simulink model "PID_SingleJoint"  (R2018b)
settings: Solver=FixedStepDiscrete  StartTime=0.0  StopTime=Inf  FixedStep=0.001  RelTol=1e-3  EnableMultiTasking=on
undefined symbols (not defined in the file): DiscIntNeverNeededParam, J1, J2, J3, J4, J5, J6, J7, Motor_Current, Motor_Position, Motor_Velocity, q, qd, Send_GUIdata, Tau
libraries: c280xlib x14, simulink x11, dspsrcs4 x6, idelinklib_common x1
(part 2 of 4)

== system PID_SingleJoint/DynamicsController/关节四正弦信号发生器 ==
  note: 0~60
  En : Inport
  q : Inport  Port=2
  Constant3 : Constant  Value=30
  Gain14 : Gain  Gain=pi/180
  Subsystem : Subsystem  mask(单关节正弦信号生产器){Freq=1/4, SimpleTime=0.001}
      mask prompts: Freq "正弦信号的频率(HZ)"; SimpleTime "正弦信号的采样时间(s)"
      mask help:
      | 采样频率不能过快，否则机械臂摆动频率也会变快，至少为1/4.
      | 采样时间只能是定时器步长的整数倍，否则会报错。
      mask Display:
      | color('red');
      | disp('单关节正弦信号发生器');
      | color('black');
      | port_label('input', 1, '外转子实际角度(rad)');
      | port_label('input', 2, '外转子正弦信号的幅值');
      | port_label('Enable','Enable')
      | port_label('output', 1, '外转子理想正弦信号');
      | port_label('output', 2, '外转子跟踪误差(rad)');
  qd : Outport
  e : Outport  Port=2
  wires:
  q/1 -> Subsystem/1(电机外转子 实际角度(rad))
  En/1 -> Subsystem/Enable
  Gain14/1 -> Subsystem/2(电机外转子 正弦信号的幅值)
  Subsystem/2(电机外转子 跟踪误差) -> e/1
  Constant3/1 -> Gain14/1
  Subsystem/1(外转子理想 正弦信号) -> qd/1

== system PID_SingleJoint/GetMotorData/CANA_284_24 ==
  note: 控制器接收ID:0x280+“ID”
  Subsystem1 : Subsystem
  eCAN Receive1 : c280xlib/eCAN Receive  chipFamily=C280x  useModule=eCAN_A  mailboxNo=24  messageID=hex2dec('284')  messageType=Standard (11-bit identifier)  sampleTime=-1  dataType=uint8  initValue=0  outputMessageLength=off  outputMessageTimeStamp=off  postInterrupt=off  interruptLine=0
      settings: SourceProductName=Embedded Coder Support Package for Texas Instruments C2000 Processors  SourceProductBaseCode=TIC2000
  wires:
  eCAN Receive1/2 -> Subsystem1/1(In1)
  eCAN Receive1/1 -> Subsystem1/Trigger

== system PID_SingleJoint/GetMotorData/CANA_285_25 ==
  note: 控制器接收ID:0x280+“ID”
  Subsystem : Subsystem
  eCAN Receive : c280xlib/eCAN Receive  chipFamily=C280x  useModule=eCAN_A  mailboxNo=25  messageID=hex2dec('285')  messageType=Standard (11-bit identifier)  sampleTime=-1  dataType=uint8  initValue=0  outputMessageLength=off  outputMessageTimeStamp=off  postInterrupt=off  interruptLine=0
      settings: SourceProductName=Embedded Coder Support Package for Texas Instruments C2000 Processors  SourceProductBaseCode=TIC2000
  wires:
  eCAN Receive/2 -> Subsystem/1(In1)
  eCAN Receive/1 -> Subsystem/Trigger

== system PID_SingleJoint/GetMotorData/CANA_286_26 ==
  note: 控制器接收ID:0x280+“ID”
  Subsystem : Subsystem
  eCAN Receive : c280xlib/eCAN Receive  chipFamily=C280x  useModule=eCAN_A  mailboxNo=26  messageID=hex2dec('286')  messageType=Standard (11-bit identifier)  sampleTime=-1  dataType=uint8  initValue=0  outputMessageLength=off  outputMessageTimeStamp=off  postInterrupt=off  interruptLine=0
      settings: SourceProductName=Embedded Coder Support Package for Texas Instruments C2000 Processors  SourceProductBaseCode=TIC2000
  wires:
  eCAN Receive/2 -> Subsystem/1(In1)
  eCAN Receive/1 -> Subsystem/Trigger

== system PID_SingleJoint/GetMotorData/CANB_281_21 ==
  note: 控制器接收ID:0x280+“ID”
  Subsystem : Subsystem
  eCAN Receive : c280xlib/eCAN Receive  chipFamily=C280x  useModule=eCAN_B  mailboxNo=21  messageID=hex2dec('281')  messageType=Standard (11-bit identifier)  sampleTime=-1  dataType=uint8  initValue=0  outputMessageLength=off  outputMessageTimeStamp=off  postInterrupt=off  interruptLine=0
      settings: SourceProductName=Embedded Coder Support Package for Texas Instruments C2000 Processors  SourceProductBaseCode=TIC2000
  wires:
  eCAN Receive/2 -> Subsystem/1(In1)
  eCAN Receive/1 -> Subsystem/Trigger

== system PID_SingleJoint/GetMotorData/CANB_282_22 ==
  note: 控制器接收ID:0x280+“ID”
  Subsystem : Subsystem
  eCAN Receive : c280xlib/eCAN Receive  chipFamily=C280x  useModule=eCAN_B  mailboxNo=22  messageID=hex2dec('282')  messageType=Standard (11-bit identifier)  sampleTime=-1  dataType=uint8  initValue=0  outputMessageLength=off  outputMessageTimeStamp=off  postInterrupt=off  interruptLine=0
      settings: SourceProductName=Embedded Coder Support Package for Texas Instruments C2000 Processors  SourceProductBaseCode=TIC2000
  wires:
  eCAN Receive/2 -> Subsystem/1(In1)
  eCAN Receive/1 -> Subsystem/Trigger

== system PID_SingleJoint/GetMotorData/CANB_283_23 ==
  note: 控制器接收ID:0x280+“ID”
  Subsystem : Subsystem
  eCAN Receive : c280xlib/eCAN Receive  chipFamily=C280x  useModule=eCAN_B  mailboxNo=23  messageID=hex2dec('283')  messageType=Standard (11-bit identifier)  sampleTime=-1  dataType=uint8  initValue=0  outputMessageLength=off  outputMessageTimeStamp=off  postInterrupt=off  interruptLine=0
      settings: SourceProductName=Embedded Coder Support Package for Texas Instruments C2000 Processors  SourceProductBaseCode=TIC2000
  wires:
  eCAN Receive/2 -> Subsystem/1(In1)
  eCAN Receive/1 -> Subsystem/Trigger

== system PID_SingleJoint/SendDataToGUI/  ==
  Enable : EnablePort
  Constant1 : Constant  Value=hex2dec('5a')  OutDataTypeStr=uint16
  Data Store Read4 : DataStoreRead  DataStoreName=Send_GUIdata
  Data Type Conversion12 : DataTypeConversion  OutDataTypeStr=uint16
  Demux : Demux  Outputs=18
  Mux : Mux  Inputs=20
  SCI Transmit : c280xlib/SCI Transmit  sciModule=A  dataHead=''  dataTail=''  postInterrupt=off  numFifo=1
      settings: SourceProductName=Embedded Coder Support Package for Texas Instruments C2000 Processors
  校验码填充 : Sum  Inputs=+++++++++++++++++++  AccumDataTypeStr=uint16
  wires:
  Demux/1 -> Mux/2, 校验码填充/2
  Mux/1 -> SCI Transmit/1
  Demux/3 -> 校验码填充/4, Mux/4
  Demux/14 -> 校验码填充/15, Mux/15
  Demux/9 -> 校验码填充/10, Mux/10
  Demux/5 -> Mux/6, 校验码填充/6
  Demux/2 -> 校验码填充/3, Mux/3
  Data Store Read4/1 -> Data Type Conversion12/1
  Demux/13 -> 校验码填充/14, Mux/14
  Demux/6 -> Mux/7, 校验码填充/7
  Demux/8 -> 校验码填充/9, Mux/9
  Demux/10 -> 校验码填充/11, Mux/11
  Demux/4 -> 校验码填充/5, Mux/5
  Demux/7 -> 校验码填充/8, Mux/8
  Demux/15 -> 校验码填充/16, Mux/16
  Demux/11 -> 校验码填充/12, Mux/12
  Demux/18 -> 校验码填充/19, Mux/19
  Demux/16 -> 校验码填充/17, Mux/17
  Constant1/1 -> 校验码填充/1, Mux/1
  Demux/17 -> 校验码填充/18, Mux/18
  校验码填充/1 -> Mux/20
  Demux/12 -> 校验码填充/13, Mux/13
  Data Type Conversion12/1 -> Demux/1

== system PID_SingleJoint/Subsystem/Model Header ==

== system PID_SingleJoint/Subsystem/Model Source ==

== system PID_SingleJoint/Subsystem/System Initialize ==

== system PID_SingleJoint/接收上位机的数据/Subsystem ==
  组号 : Inport
  数据 : Inport  Port=2
  Enable : EnablePort
  Joint1 : Subsystem  TreatAsAtomicUnit=on
  Joint2 : Subsystem  TreatAsAtomicUnit=on
  Joint3 : Subsystem  TreatAsAtomicUnit=on
  Joint4 : Subsystem  TreatAsAtomicUnit=on
  Joint5 : Subsystem  TreatAsAtomicUnit=on
  Joint6 : Subsystem  TreatAsAtomicUnit=on
  Joint7 : Subsystem  TreatAsAtomicUnit=on
  Switch Case : SwitchCase  CaseConditions={1 2 3 4 5 6 7}  ShowDefaultCase=off
  wires:
  数据/1 -> Joint7/1(Joint7), Joint5/1(Joint5), Joint4/1(Joint4), Joint3/1(Joint3), Joint2/1(Joint2), Joint1/1(Joint1), Joint6/1(Joint6)
  Switch Case/5 -> Joint5/Action
  Switch Case/6 -> Joint6/Action
  Switch Case/2 -> Joint2/Action
  Switch Case/1 -> Joint1/Action
  Switch Case/3 -> Joint3/Action
  Switch Case/4 -> Joint4/Action
  组号/1 -> Switch Case/1
  Switch Case/7 -> Joint7/Action

== system PID_SingleJoint/接收上位机的数据/获取用户命令 ==
  " " : c280xlib/SCI Receive  sciModule=A  dataHead=''  dataTail=''  dataType=uint16  dataDim=9  initValue=0  errOption=Output the last received value  errValue=0  sampleTime=-1  outputStatus=on  postInterrupt=off  numFifo=1
      settings: SourceProductName=Embedded Coder Support Package for Texas Instruments C2000 Processors  SourceProductBaseCode=TIC2000
  Constant : Constant  Value=false  OutDataTypeStr=boolean
  Constant1 : Constant  Value=true  OutDataTypeStr=boolean
  Data Store Write1 : DataStoreWrite  DataStoreName=PTX
  Logical Operator : Logic  AllPortsSameDT=off  OutDataTypeStr=boolean
  Switch : Switch  Criteria=u2 > Threshold
  消息校验 : Subsystem
  消息 : Outport
  wires:
  消息校验/2(使能) -> Logical Operator/1
  Switch/1 -> Logical Operator/2
  Constant1/1 -> Switch/3
  " "/2 -> Switch/2
  消息校验/1(消息) -> 消息/1
  " "/1 -> 消息校验/1(数据)
  Logical Operator/1 -> Data Store Write1/1
  Constant/1 -> Switch/1

== system PID_SingleJoint/DynamicsController/DriveMotor/BottomDriver ==
  JOINT1 : Inport
  JOINT2 : Inport  Port=2
  JOINT3 : Inport  Port=3
  JOINT4 : Inport  Port=4
  JOINT5 : Inport  Port=5
  JOINT6 : Inport  Port=6
  Enable : EnablePort
  Constant : Constant  Value=0  OutDataTypeStr=uint8
  Data Store Write : DataStoreWrite  DataStoreName=TXD
  Joint1 : Subsystem  Priority=1  Commented=on
  Joint2 : Subsystem  Priority=2  Commented=on
  Joint3 : Subsystem  Priority=3  Commented=on
  Joint4 : Subsystem  Priority=4  Commented=on
  Joint5 : Subsystem  Priority=5
  Joint6 : Subsystem  Priority=6  Commented=on
  wires:
  JOINT3/1 -> Joint3/1(In1)
  JOINT5/1 -> Joint5/1(In1)
  JOINT2/1 -> Joint2/1(In1)
  JOINT4/1 -> Joint4/1(In1)
  JOINT6/1 -> Joint6/1(In1)
  JOINT1/1 -> Joint1/1(In6)
  Constant/1 -> Data Store Write/1

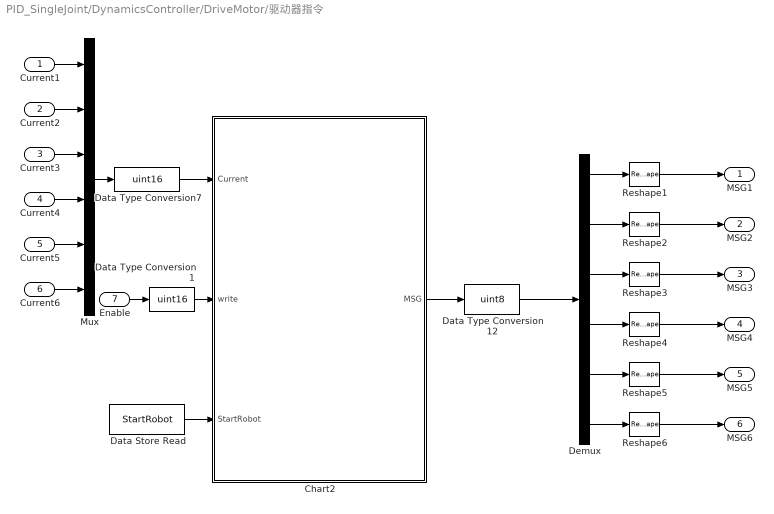
== system PID_SingleJoint/DynamicsController/DriveMotor/驱动器指令 ==
  Current1 : Inport
  Current2 : Inport  Port=2
  Current3 : Inport  Port=3
  Current4 : Inport  Port=4
  Current5 : Inport  Port=5
  Current6 : Inport  Port=6
  Enable : Inport  Port=7
  Chart2 : Stateflow chart  TreatAsAtomicUnit=on
  Data Store Read : DataStoreRead  DataStoreName=StartRobot
  Data Type Conversion1 : DataTypeConversion  OutDataTypeStr=uint16
  Data Type Conversion12 : DataTypeConversion  OutDataTypeStr=uint8
  Data Type Conversion7 : DataTypeConversion  OutDataTypeStr=uint16
  Demux : Demux  Outputs=6
  Mux : Mux  Inputs=6
  Reshape{1..6} (6 alike) : Reshape  OutputDimensionality=Customize  OutputDimensions=[1,8]
  MSG1 : Outport
  MSG2 : Outport  Port=2
  MSG3 : Outport  Port=3
  MSG4 : Outport  Port=4
  MSG5 : Outport  Port=5
  MSG6 : Outport  Port=6
  wires:
  Data Store Read/1 -> Chart2/3(StartRobot)
  Current1/1 -> Mux/1
  Current2/1 -> Mux/2
  Current3/1 -> Mux/3
  Current4/1 -> Mux/4
  Current5/1 -> Mux/5
  Current6/1 -> Mux/6
  Mux/1 -> Data Type Conversion7/1
  Enable/1 -> Data Type Conversion1/1
  Data Type Conversion7/1 -> Chart2/1(Current)
  Demux/5 -> Reshape5/1
  Demux/4 -> Reshape4/1
  Demux/6 -> Reshape6/1
  Demux/3 -> Reshape3/1
  Demux/2 -> Reshape2/1
  Demux/1 -> Reshape1/1
  Data Type Conversion12/1 -> Demux/1
  Chart2/1(MSG) -> Data Type Conversion12/1
  Reshape1/1 -> MSG1/1
  Reshape2/1 -> MSG2/1
  Reshape3/1 -> MSG3/1
  Reshape4/1 -> MSG4/1
  Reshape5/1 -> MSG5/1
  Reshape6/1 -> MSG6/1
  Data Type Conversion1/1 -> Chart2/2(write)

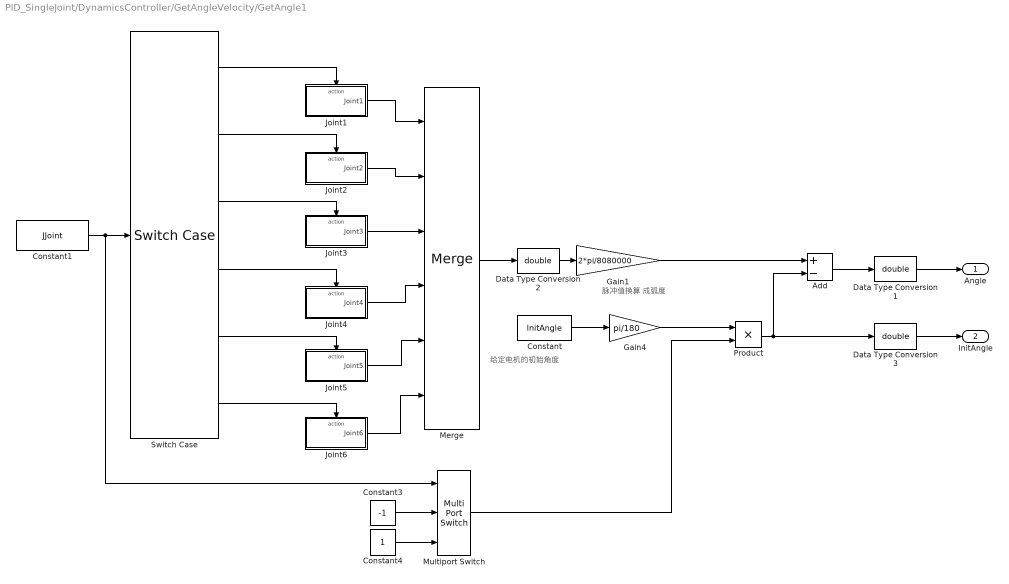
== system PID_SingleJoint/DynamicsController/GetAngleVelocity/GetAngle1 ==
  note: 脉冲值换算
      | 成弧度
  note: 给定电机的初始角度
  Add : Sum  Inputs=+-
  Constant : Constant  Value=InitAngle
  Constant1 : Constant  Value=JJoint  OutDataTypeStr=uint8
  Constant3 : Constant  Value=-1
  Constant4 : Constant
  Data Type Conversion1 : DataTypeConversion  OutDataTypeStr=double
  Data Type Conversion2 : DataTypeConversion  OutDataTypeStr=double
  Data Type Conversion3 : DataTypeConversion  OutDataTypeStr=double
  Gain1 : Gain  Gain=2*pi/8080000
  Gain4 : Gain  Gain=pi/180
  Joint1 : Subsystem  TreatAsAtomicUnit=on
  Joint2 : Subsystem  TreatAsAtomicUnit=on
  Joint3 : Subsystem  TreatAsAtomicUnit=on
  Joint4 : Subsystem  TreatAsAtomicUnit=on
  Joint5 : Subsystem  TreatAsAtomicUnit=on
  Joint6 : Subsystem  TreatAsAtomicUnit=on
  Merge : Merge  Inputs=6  InitialOutput=0
  Multiport Switch : MultiPortSwitch  DataPortOrder=Specify indices  Inputs=2  DataPortIndices={3,[1,2,4,5,6]}
  Product : Product
  Switch Case : SwitchCase  CaseConditions={1 2 3 4 5 6}  ShowDefaultCase=off
  Angle : Outport
  InitAngle : Outport  Port=2
  wires:
  Data Type Conversion2/1 -> Gain1/1
  Data Type Conversion1/1 -> Angle/1
  Joint6/1(Joint6) -> Merge/6
  Joint5/1(Joint5) -> Merge/5
  Joint4/1(Joint4) -> Merge/4
  Joint3/1(Joint3) -> Merge/3
  Joint2/1(Joint2) -> Merge/2
  Joint1/1(Joint1) -> Merge/1
  Switch Case/6 -> Joint6/Action
  Switch Case/5 -> Joint5/Action
  Switch Case/4 -> Joint4/Action
  Switch Case/3 -> Joint3/Action
  Switch Case/2 -> Joint2/Action
  Switch Case/1 -> Joint1/Action
  Constant/1 -> Gain4/1
  Add/1 -> Data Type Conversion1/1
  Gain1/1 -> Add/1
  Gain4/1 -> Product/1
  Merge/1 -> Data Type Conversion2/1
  Multiport Switch/1 -> Product/2
  Constant4/1 -> Multiport Switch/3
  Constant3/1 -> Multiport Switch/2
  Constant1/1 -> Multiport Switch/1, Switch Case/1
  Product/1 -> Data Type Conversion3/1, Add/2
  Data Type Conversion3/1 -> InitAngle/1

== system PID_SingleJoint/DynamicsController/GetAngleVelocity/GetAngle2 ==
  note: 给定电机的初始角度
  note: 脉冲值换算
      | 成弧度
  Add : Sum  Inputs=+-
  Constant : Constant  Value=InitAngle
  Constant1 : Constant  Value=JJoint  OutDataTypeStr=uint8
  Constant3 : Constant  Value=-1
  Constant4 : Constant
  Data Type Conversion1 : DataTypeConversion  OutDataTypeStr=double
  Data Type Conversion2 : DataTypeConversion  OutDataTypeStr=double
  Data Type Conversion3 : DataTypeConversion  OutDataTypeStr=double
  Gain1 : Gain  Gain=2*pi/8080000
  Gain4 : Gain  Gain=pi/180
  Joint1 : Subsystem  TreatAsAtomicUnit=on
  Joint2 : Subsystem  TreatAsAtomicUnit=on
  Joint3 : Subsystem  TreatAsAtomicUnit=on
  Joint4 : Subsystem  TreatAsAtomicUnit=on
  Joint5 : Subsystem  TreatAsAtomicUnit=on
  Joint6 : Subsystem  TreatAsAtomicUnit=on
  Merge : Merge  Inputs=6  InitialOutput=0
  Multiport Switch : MultiPortSwitch  DataPortOrder=Specify indices  Inputs=2  DataPortIndices={3,[1,2,4,5,6]}
  Product : Product
  Switch Case : SwitchCase  CaseConditions={1 2 3 4 5 6}  ShowDefaultCase=off
  Angle : Outport
  InitAngle : Outport  Port=2
  wires:
  Data Type Conversion3/1 -> InitAngle/1
  Product/1 -> Add/2, Data Type Conversion3/1
  Constant1/1 -> Switch Case/1, Multiport Switch/1
  Constant3/1 -> Multiport Switch/2
  Constant4/1 -> Multiport Switch/3
  Multiport Switch/1 -> Product/2
  Merge/1 -> Data Type Conversion2/1
  Gain4/1 -> Product/1
  Gain1/1 -> Add/1
  Add/1 -> Data Type Conversion1/1
  Constant/1 -> Gain4/1
  Switch Case/1 -> Joint1/Action
  Switch Case/2 -> Joint2/Action
  Switch Case/3 -> Joint3/Action
  Switch Case/4 -> Joint4/Action
  Switch Case/5 -> Joint5/Action
  Switch Case/6 -> Joint6/Action
  Joint1/1(Joint1) -> Merge/1
  Joint2/1(Joint2) -> Merge/2
  Joint3/1(Joint3) -> Merge/3
  Joint4/1(Joint4) -> Merge/4
  Joint5/1(Joint5) -> Merge/5
  Joint6/1(Joint6) -> Merge/6
  Data Type Conversion1/1 -> Angle/1
  Data Type Conversion2/1 -> Gain1/1

== system PID_SingleJoint/DynamicsController/GetAngleVelocity/GetAngle3 ==
  note: 脉冲值换算
      | 成弧度
  note: 给定电机的初始角度
  Add : Sum  Inputs=+-
  Constant : Constant  Value=InitAngle
  Constant1 : Constant  Value=JJoint  OutDataTypeStr=uint8
  Constant3 : Constant  Value=-1
  Constant4 : Constant
  Data Type Conversion1 : DataTypeConversion  OutDataTypeStr=double
  Data Type Conversion2 : DataTypeConversion  OutDataTypeStr=double
  Data Type Conversion3 : DataTypeConversion  OutDataTypeStr=double
  Gain1 : Gain  Gain=2*pi/8080000
  Gain4 : Gain  Gain=pi/180
  Joint1 : Subsystem  TreatAsAtomicUnit=on
  Joint2 : Subsystem  TreatAsAtomicUnit=on
  Joint3 : Subsystem  TreatAsAtomicUnit=on
  Joint4 : Subsystem  TreatAsAtomicUnit=on
  Joint5 : Subsystem  TreatAsAtomicUnit=on
  Joint6 : Subsystem  TreatAsAtomicUnit=on
  Merge : Merge  Inputs=6  InitialOutput=0
  Multiport Switch : MultiPortSwitch  DataPortOrder=Specify indices  Inputs=2  DataPortIndices={3,[1,2,4,5,6]}
  Product : Product
  Switch Case : SwitchCase  CaseConditions={1 2 3 4 5 6}  ShowDefaultCase=off
  Angle : Outport
  InitAngle : Outport  Port=2
  wires:
  Data Type Conversion2/1 -> Gain1/1
  Data Type Conversion1/1 -> Angle/1
  Joint6/1(Joint6) -> Merge/6
  Joint5/1(Joint5) -> Merge/5
  Joint4/1(Joint4) -> Merge/4
  Joint3/1(Joint3) -> Merge/3
  Joint2/1(Joint2) -> Merge/2
  Joint1/1(Joint1) -> Merge/1
  Switch Case/6 -> Joint6/Action
  Switch Case/5 -> Joint5/Action
  Switch Case/4 -> Joint4/Action
  Switch Case/3 -> Joint3/Action
  Switch Case/2 -> Joint2/Action
  Switch Case/1 -> Joint1/Action
  Constant/1 -> Gain4/1
  Add/1 -> Data Type Conversion1/1
  Gain1/1 -> Add/1
  Gain4/1 -> Product/1
  Merge/1 -> Data Type Conversion2/1
  Multiport Switch/1 -> Product/2
  Constant4/1 -> Multiport Switch/3
  Constant3/1 -> Multiport Switch/2
  Constant1/1 -> Multiport Switch/1, Switch Case/1
  Product/1 -> Data Type Conversion3/1, Add/2
  Data Type Conversion3/1 -> InitAngle/1

== system PID_SingleJoint/DynamicsController/GetAngleVelocity/GetAngle4 ==
  note: 给定电机的初始角度
  note: 脉冲值换算
      | 成弧度
  Add : Sum  Inputs=+-
  Constant : Constant  Value=InitAngle
  Constant1 : Constant  Value=JJoint  OutDataTypeStr=uint8
  Constant3 : Constant  Value=-1
  Constant4 : Constant
  Data Type Conversion1 : DataTypeConversion  OutDataTypeStr=double
  Data Type Conversion2 : DataTypeConversion  OutDataTypeStr=double
  Data Type Conversion3 : DataTypeConversion  OutDataTypeStr=double
  Gain1 : Gain  Gain=2*pi/8080000
  Gain4 : Gain  Gain=pi/180
  Joint1 : Subsystem  TreatAsAtomicUnit=on
  Joint2 : Subsystem  TreatAsAtomicUnit=on
  Joint3 : Subsystem  TreatAsAtomicUnit=on
  Joint4 : Subsystem  TreatAsAtomicUnit=on
  Joint5 : Subsystem  TreatAsAtomicUnit=on
  Joint6 : Subsystem  TreatAsAtomicUnit=on
  Merge : Merge  Inputs=6  InitialOutput=0
  Multiport Switch : MultiPortSwitch  DataPortOrder=Specify indices  Inputs=2  DataPortIndices={3,[1,2,4,5,6]}
  Product : Product
  Switch Case : SwitchCase  CaseConditions={1 2 3 4 5 6}  ShowDefaultCase=off
  Angle : Outport
  InitAngle : Outport  Port=2
  wires:
  Data Type Conversion3/1 -> InitAngle/1
  Product/1 -> Add/2, Data Type Conversion3/1
  Constant1/1 -> Switch Case/1, Multiport Switch/1
  Constant3/1 -> Multiport Switch/2
  Constant4/1 -> Multiport Switch/3
  Multiport Switch/1 -> Product/2
  Merge/1 -> Data Type Conversion2/1
  Gain4/1 -> Product/1
  Gain1/1 -> Add/1
  Add/1 -> Data Type Conversion1/1
  Constant/1 -> Gain4/1
  Switch Case/1 -> Joint1/Action
  Switch Case/2 -> Joint2/Action
  Switch Case/3 -> Joint3/Action
  Switch Case/4 -> Joint4/Action
  Switch Case/5 -> Joint5/Action
  Switch Case/6 -> Joint6/Action
  Joint1/1(Joint1) -> Merge/1
  Joint2/1(Joint2) -> Merge/2
  Joint3/1(Joint3) -> Merge/3
  Joint4/1(Joint4) -> Merge/4
  Joint5/1(Joint5) -> Merge/5
  Joint6/1(Joint6) -> Merge/6
  Data Type Conversion1/1 -> Angle/1
  Data Type Conversion2/1 -> Gain1/1

== system PID_SingleJoint/DynamicsController/GetAngleVelocity/GetAngle5 ==
  note: 脉冲值换算
      | 成弧度
  note: 给定电机的初始角度
  Add : Sum  Inputs=+-
  Constant : Constant  Value=InitAngle
  Constant1 : Constant  Value=JJoint  OutDataTypeStr=uint8
  Constant3 : Constant  Value=-1
  Constant4 : Constant
  Data Type Conversion1 : DataTypeConversion  OutDataTypeStr=double
  Data Type Conversion2 : DataTypeConversion  OutDataTypeStr=double
  Data Type Conversion3 : DataTypeConversion  OutDataTypeStr=double
  Gain1 : Gain  Gain=2*pi/8080000
  Gain4 : Gain  Gain=pi/180
  Joint1 : Subsystem  TreatAsAtomicUnit=on
  Joint2 : Subsystem  TreatAsAtomicUnit=on
  Joint3 : Subsystem  TreatAsAtomicUnit=on
  Joint4 : Subsystem  TreatAsAtomicUnit=on
  Joint5 : Subsystem  TreatAsAtomicUnit=on
  Joint6 : Subsystem  TreatAsAtomicUnit=on
  Merge : Merge  Inputs=6  InitialOutput=0
  Multiport Switch : MultiPortSwitch  DataPortOrder=Specify indices  Inputs=2  DataPortIndices={3,[1,2,4,5,6]}
  Product : Product
  Switch Case : SwitchCase  CaseConditions={1 2 3 4 5 6}  ShowDefaultCase=off
  Angle : Outport
  InitAngle : Outport  Port=2
  wires:
  Data Type Conversion2/1 -> Gain1/1
  Data Type Conversion1/1 -> Angle/1
  Joint6/1(Joint6) -> Merge/6
  Joint5/1(Joint5) -> Merge/5
  Joint4/1(Joint4) -> Merge/4
  Joint3/1(Joint3) -> Merge/3
  Joint2/1(Joint2) -> Merge/2
  Joint1/1(Joint1) -> Merge/1
  Switch Case/6 -> Joint6/Action
  Switch Case/5 -> Joint5/Action
  Switch Case/4 -> Joint4/Action
  Switch Case/3 -> Joint3/Action
  Switch Case/2 -> Joint2/Action
  Switch Case/1 -> Joint1/Action
  Constant/1 -> Gain4/1
  Add/1 -> Data Type Conversion1/1
  Gain1/1 -> Add/1
  Gain4/1 -> Product/1
  Merge/1 -> Data Type Conversion2/1
  Multiport Switch/1 -> Product/2
  Constant4/1 -> Multiport Switch/3
  Constant3/1 -> Multiport Switch/2
  Constant1/1 -> Multiport Switch/1, Switch Case/1
  Product/1 -> Data Type Conversion3/1, Add/2
  Data Type Conversion3/1 -> InitAngle/1

== system PID_SingleJoint/DynamicsController/GetAngleVelocity/GetAngle6 ==
  note: 给定电机的初始角度
  note: 脉冲值换算
      | 成弧度
  Add : Sum  Inputs=+-
  Constant : Constant  Value=InitAngle
  Constant1 : Constant  Value=JJoint  OutDataTypeStr=uint8
  Constant3 : Constant  Value=-1
  Constant4 : Constant
  Data Type Conversion1 : DataTypeConversion  OutDataTypeStr=double
  Data Type Conversion2 : DataTypeConversion  OutDataTypeStr=double
  Data Type Conversion3 : DataTypeConversion  OutDataTypeStr=double
  Gain1 : Gain  Gain=2*pi/8080000
  Gain4 : Gain  Gain=pi/180
  Joint1 : Subsystem  TreatAsAtomicUnit=on
  Joint2 : Subsystem  TreatAsAtomicUnit=on
  Joint3 : Subsystem  TreatAsAtomicUnit=on
  Joint4 : Subsystem  TreatAsAtomicUnit=on
  Joint5 : Subsystem  TreatAsAtomicUnit=on
  Joint6 : Subsystem  TreatAsAtomicUnit=on
  Merge : Merge  Inputs=6  InitialOutput=0
  Multiport Switch : MultiPortSwitch  DataPortOrder=Specify indices  Inputs=2  DataPortIndices={3,[1,2,4,5,6]}
  Product : Product
  Switch Case : SwitchCase  CaseConditions={1 2 3 4 5 6}  ShowDefaultCase=off
  Angle : Outport
  InitAngle : Outport  Port=2
  wires:
  Data Type Conversion3/1 -> InitAngle/1
  Product/1 -> Add/2, Data Type Conversion3/1
  Constant1/1 -> Switch Case/1, Multiport Switch/1
  Constant3/1 -> Multiport Switch/2
  Constant4/1 -> Multiport Switch/3
  Multiport Switch/1 -> Product/2
  Merge/1 -> Data Type Conversion2/1
  Gain4/1 -> Product/1
  Gain1/1 -> Add/1
  Add/1 -> Data Type Conversion1/1
  Constant/1 -> Gain4/1
  Switch Case/1 -> Joint1/Action
  Switch Case/2 -> Joint2/Action
  Switch Case/3 -> Joint3/Action
  Switch Case/4 -> Joint4/Action
  Switch Case/5 -> Joint5/Action
  Switch Case/6 -> Joint6/Action
  Joint1/1(Joint1) -> Merge/1
  Joint2/1(Joint2) -> Merge/2
  Joint3/1(Joint3) -> Merge/3
  Joint4/1(Joint4) -> Merge/4
  Joint5/1(Joint5) -> Merge/5
  Joint6/1(Joint6) -> Merge/6
  Data Type Conversion1/1 -> Angle/1
  Data Type Conversion2/1 -> Gain1/1

== system PID_SingleJoint/DynamicsController/GetAngleVelocity/GetAngleSpeed ==
  note: 换算成角速度2π/1min
  Constant1 : Constant  Value=JJoint
  Data Type Conversion3 : DataTypeConversion  OutDataTypeStr=double
  Gain3 : Gain  Gain=2*pi/60
  Gain9 : Gain  Gain=1/101
  Joint1 : Subsystem  TreatAsAtomicUnit=on
  Joint2 : Subsystem  TreatAsAtomicUnit=on
  Joint3 : Subsystem  TreatAsAtomicUnit=on
  Joint4 : Subsystem  TreatAsAtomicUnit=on
  Joint5 : Subsystem  TreatAsAtomicUnit=on
  Joint6 : Subsystem  TreatAsAtomicUnit=on
  Merge1 : Merge  Inputs=6  InitialOutput=0
  Switch Case : SwitchCase  CaseConditions={1 2 3 4 5 6}  ShowDefaultCase=off
  Velcity : Outport
  wires:
  Constant1/1 -> Switch Case/1
  Switch Case/1 -> Joint1/Action
  Switch Case/2 -> Joint2/Action
  Switch Case/3 -> Joint3/Action
  Switch Case/4 -> Joint4/Action
  Switch Case/5 -> Joint5/Action
  Switch Case/6 -> Joint6/Action
  Data Type Conversion3/1 -> Gain3/1
  Joint6/1(Joint6_Velocity) -> Merge1/6
  Joint5/1(Joint5_Velocity) -> Merge1/5
  Joint4/1(Joint4_Velocity) -> Merge1/4
  Joint3/1(Joint3_Velocity) -> Merge1/3
  Joint2/1(Joint2_Velocity) -> Merge1/2
  Joint1/1(Joint1_Velocity) -> Merge1/1
  Gain3/1 -> Gain9/1
  Gain9/1 -> Velcity/1
  Merge1/1 -> Data Type Conversion3/1

== system PID_SingleJoint/DynamicsController/GetAngleVelocity/GetAngleSpeed1 ==
  note: 换算成角速度2π/1min
  Constant1 : Constant  Value=JJoint
  Data Type Conversion3 : DataTypeConversion  OutDataTypeStr=double
  Gain3 : Gain  Gain=2*pi/60
  Gain9 : Gain  Gain=1/101
  Joint1 : Subsystem  TreatAsAtomicUnit=on
  Joint2 : Subsystem  TreatAsAtomicUnit=on
  Joint3 : Subsystem  TreatAsAtomicUnit=on
  Joint4 : Subsystem  TreatAsAtomicUnit=on
  Joint5 : Subsystem  TreatAsAtomicUnit=on
  Joint6 : Subsystem  TreatAsAtomicUnit=on
  Merge1 : Merge  Inputs=6  InitialOutput=0
  Switch Case : SwitchCase  CaseConditions={1 2 3 4 5 6}  ShowDefaultCase=off
  Velcity : Outport
  wires:
  Merge1/1 -> Data Type Conversion3/1
  Gain9/1 -> Velcity/1
  Gain3/1 -> Gain9/1
  Joint1/1(Joint1_Velocity) -> Merge1/1
  Joint2/1(Joint2_Velocity) -> Merge1/2
  Joint3/1(Joint3_Velocity) -> Merge1/3
  Joint4/1(Joint4_Velocity) -> Merge1/4
  Joint5/1(Joint5_Velocity) -> Merge1/5
  Joint6/1(Joint6_Velocity) -> Merge1/6
  Data Type Conversion3/1 -> Gain3/1
  Switch Case/6 -> Joint6/Action
  Switch Case/5 -> Joint5/Action
  Switch Case/4 -> Joint4/Action
  Switch Case/3 -> Joint3/Action
  Switch Case/2 -> Joint2/Action
  Switch Case/1 -> Joint1/Action
  Constant1/1 -> Switch Case/1

== system PID_SingleJoint/DynamicsController/GetAngleVelocity/GetAngleSpeed2 ==
  note: 换算成角速度2π/1min
  Constant1 : Constant  Value=JJoint
  Data Type Conversion3 : DataTypeConversion  OutDataTypeStr=double
  Gain3 : Gain  Gain=2*pi/60
  Gain9 : Gain  Gain=1/101
  Joint1 : Subsystem  TreatAsAtomicUnit=on
  Joint2 : Subsystem  TreatAsAtomicUnit=on
  Joint3 : Subsystem  TreatAsAtomicUnit=on
  Joint4 : Subsystem  TreatAsAtomicUnit=on
  Joint5 : Subsystem  TreatAsAtomicUnit=on
  Joint6 : Subsystem  TreatAsAtomicUnit=on
  Merge1 : Merge  Inputs=6  InitialOutput=0
  Switch Case : SwitchCase  CaseConditions={1 2 3 4 5 6}  ShowDefaultCase=off
  Velcity : Outport
  wires:
  Constant1/1 -> Switch Case/1
  Switch Case/1 -> Joint1/Action
  Switch Case/2 -> Joint2/Action
  Switch Case/3 -> Joint3/Action
  Switch Case/4 -> Joint4/Action
  Switch Case/5 -> Joint5/Action
  Switch Case/6 -> Joint6/Action
  Data Type Conversion3/1 -> Gain3/1
  Joint6/1(Joint6_Velocity) -> Merge1/6
  Joint5/1(Joint5_Velocity) -> Merge1/5
  Joint4/1(Joint4_Velocity) -> Merge1/4
  Joint3/1(Joint3_Velocity) -> Merge1/3
  Joint2/1(Joint2_Velocity) -> Merge1/2
  Joint1/1(Joint1_Velocity) -> Merge1/1
  Gain3/1 -> Gain9/1
  Gain9/1 -> Velcity/1
  Merge1/1 -> Data Type Conversion3/1

== system PID_SingleJoint/DynamicsController/GetAngleVelocity/GetAngleSpeed3 ==
  note: 换算成角速度2π/1min
  Constant1 : Constant  Value=JJoint
  Data Type Conversion3 : DataTypeConversion  OutDataTypeStr=double
  Gain3 : Gain  Gain=2*pi/60
  Gain9 : Gain  Gain=1/101
  Joint1 : Subsystem  TreatAsAtomicUnit=on
  Joint2 : Subsystem  TreatAsAtomicUnit=on
  Joint3 : Subsystem  TreatAsAtomicUnit=on
  Joint4 : Subsystem  TreatAsAtomicUnit=on
  Joint5 : Subsystem  TreatAsAtomicUnit=on
  Joint6 : Subsystem  TreatAsAtomicUnit=on
  Merge1 : Merge  Inputs=6  InitialOutput=0
  Switch Case : SwitchCase  CaseConditions={1 2 3 4 5 6}  ShowDefaultCase=off
  Velcity : Outport
  wires:
  Merge1/1 -> Data Type Conversion3/1
  Gain9/1 -> Velcity/1
  Gain3/1 -> Gain9/1
  Joint1/1(Joint1_Velocity) -> Merge1/1
  Joint2/1(Joint2_Velocity) -> Merge1/2
  Joint3/1(Joint3_Velocity) -> Merge1/3
  Joint4/1(Joint4_Velocity) -> Merge1/4
  Joint5/1(Joint5_Velocity) -> Merge1/5
  Joint6/1(Joint6_Velocity) -> Merge1/6
  Data Type Conversion3/1 -> Gain3/1
  Switch Case/6 -> Joint6/Action
  Switch Case/5 -> Joint5/Action
  Switch Case/4 -> Joint4/Action
  Switch Case/3 -> Joint3/Action
  Switch Case/2 -> Joint2/Action
  Switch Case/1 -> Joint1/Action
  Constant1/1 -> Switch Case/1

== system PID_SingleJoint/DynamicsController/GetAngleVelocity/GetAngleSpeed4 ==
  note: 换算成角速度2π/1min
  Constant1 : Constant  Value=JJoint
  Data Type Conversion3 : DataTypeConversion  OutDataTypeStr=double
  Gain3 : Gain  Gain=2*pi/60
  Gain9 : Gain  Gain=1/101
  Joint1 : Subsystem  TreatAsAtomicUnit=on
  Joint2 : Subsystem  TreatAsAtomicUnit=on
  Joint3 : Subsystem  TreatAsAtomicUnit=on
  Joint4 : Subsystem  TreatAsAtomicUnit=on
  Joint5 : Subsystem  TreatAsAtomicUnit=on
  Joint6 : Subsystem  TreatAsAtomicUnit=on
  Merge1 : Merge  Inputs=6  InitialOutput=0
  Switch Case : SwitchCase  CaseConditions={1 2 3 4 5 6}  ShowDefaultCase=off
  Velcity : Outport
  wires:
  Constant1/1 -> Switch Case/1
  Switch Case/1 -> Joint1/Action
  Switch Case/2 -> Joint2/Action
  Switch Case/3 -> Joint3/Action
  Switch Case/4 -> Joint4/Action
  Switch Case/5 -> Joint5/Action
  Switch Case/6 -> Joint6/Action
  Data Type Conversion3/1 -> Gain3/1
  Joint6/1(Joint6_Velocity) -> Merge1/6
  Joint5/1(Joint5_Velocity) -> Merge1/5
  Joint4/1(Joint4_Velocity) -> Merge1/4
  Joint3/1(Joint3_Velocity) -> Merge1/3
  Joint2/1(Joint2_Velocity) -> Merge1/2
  Joint1/1(Joint1_Velocity) -> Merge1/1
  Gain3/1 -> Gain9/1
  Gain9/1 -> Velcity/1
  Merge1/1 -> Data Type Conversion3/1

== system PID_SingleJoint/DynamicsController/GetAngleVelocity/GetAngleSpeed5 ==
  note: 换算成角速度2π/1min
  Constant1 : Constant  Value=JJoint
  Data Type Conversion3 : DataTypeConversion  OutDataTypeStr=double
  Gain3 : Gain  Gain=2*pi/60
  Gain9 : Gain  Gain=1/101
  Joint1 : Subsystem  TreatAsAtomicUnit=on
  Joint2 : Subsystem  TreatAsAtomicUnit=on
  Joint3 : Subsystem  TreatAsAtomicUnit=on
  Joint4 : Subsystem  TreatAsAtomicUnit=on
  Joint5 : Subsystem  TreatAsAtomicUnit=on
  Joint6 : Subsystem  TreatAsAtomicUnit=on
  Merge1 : Merge  Inputs=6  InitialOutput=0
  Switch Case : SwitchCase  CaseConditions={1 2 3 4 5 6}  ShowDefaultCase=off
  Velcity : Outport
  wires:
  Merge1/1 -> Data Type Conversion3/1
  Gain9/1 -> Velcity/1
  Gain3/1 -> Gain9/1
  Joint1/1(Joint1_Velocity) -> Merge1/1
  Joint2/1(Joint2_Velocity) -> Merge1/2
  Joint3/1(Joint3_Velocity) -> Merge1/3
  Joint4/1(Joint4_Velocity) -> Merge1/4
  Joint5/1(Joint5_Velocity) -> Merge1/5
  Joint6/1(Joint6_Velocity) -> Merge1/6
  Data Type Conversion3/1 -> Gain3/1
  Switch Case/6 -> Joint6/Action
  Switch Case/5 -> Joint5/Action
  Switch Case/4 -> Joint4/Action
  Switch Case/3 -> Joint3/Action
  Switch Case/2 -> Joint2/Action
  Switch Case/1 -> Joint1/Action
  Constant1/1 -> Switch Case/1

== system PID_SingleJoint/DynamicsController/PID_Controller/PID_Controller1 ==
  error : Inport
  KP : Inport  Port=2
  KI : Inport  Port=3
  KD : Inport  Port=4
  Data Type Conversion{1..4} (4 alike) : DataTypeConversion  OutDataTypeStr=double
  Discrete Derivative1 : simulink/Discrete/Discrete Derivative  gainval=1.0  ICPrevScaledInput=0.0  OutMin=[]  OutMax=[]  OutDataType=fixdt(1, 16)  OutScaling=2^-10  DoSatur=off
  Discrete-Time Integrator : DiscreteIntegrator  SampleTime=-1  LimitOutput=on  UpperSaturationLimit=1000  LowerSaturationLimit=-1000  ICPrevOutput=DiscIntNeverNeededParam  ICPrevScaledInput=DiscIntNeverNeededParam
  Product1 : Product
  Product2 : Product
  Product3 : Product
  Sum1 : Sum  Inputs=+++
  Tau : Outport
  wires:
  Product2/1 -> Discrete-Time Integrator/1
  error/1 -> Data Type Conversion1/1
  Product3/1 -> Discrete Derivative1/1
  KP/1 -> Data Type Conversion3/1
  Sum1/1 -> Tau/1
  Discrete Derivative1/1 -> Sum1/3
  Product1/1 -> Sum1/1
  Discrete-Time Integrator/1 -> Sum1/2
  KI/1 -> Data Type Conversion2/1
  KD/1 -> Data Type Conversion4/1
  Data Type Conversion3/1 -> Product1/1
  Data Type Conversion1/1 -> Product1/2, Product3/1, Product2/1
  Data Type Conversion2/1 -> Product2/2
  Data Type Conversion4/1 -> Product3/2

== system PID_SingleJoint/DynamicsController/PID_Controller/PID_Controller2 ==
  error : Inport
  KP : Inport  Port=2
  KI : Inport  Port=3
  KD : Inport  Port=4
  Data Type Conversion{1..4} (4 alike) : DataTypeConversion  OutDataTypeStr=double
  Discrete Derivative1 : simulink/Discrete/Discrete Derivative  gainval=1.0  ICPrevScaledInput=0.0  OutMin=[]  OutMax=[]  OutDataType=fixdt(1, 16)  OutScaling=2^-10  DoSatur=off
  Discrete-Time Integrator : DiscreteIntegrator  SampleTime=-1  LimitOutput=on  UpperSaturationLimit=1000  LowerSaturationLimit=-1000  ICPrevOutput=DiscIntNeverNeededParam  ICPrevScaledInput=DiscIntNeverNeededParam
  Product1 : Product
  Product2 : Product
  Product3 : Product
  Sum1 : Sum  Inputs=+++
  Tau : Outport
  wires:
  Data Type Conversion4/1 -> Product3/2
  Data Type Conversion2/1 -> Product2/2
  Data Type Conversion1/1 -> Product2/1, Product3/1, Product1/2
  Data Type Conversion3/1 -> Product1/1
  KD/1 -> Data Type Conversion4/1
  KI/1 -> Data Type Conversion2/1
  Discrete-Time Integrator/1 -> Sum1/2
  Product1/1 -> Sum1/1
  Discrete Derivative1/1 -> Sum1/3
  Sum1/1 -> Tau/1
  KP/1 -> Data Type Conversion3/1
  Product3/1 -> Discrete Derivative1/1
  error/1 -> Data Type Conversion1/1
  Product2/1 -> Discrete-Time Integrator/1

== system PID_SingleJoint/DynamicsController/PID_Controller/PID_Controller3 ==
  error : Inport
  KP : Inport  Port=2
  KI : Inport  Port=3
  KD : Inport  Port=4
  Data Type Conversion{1..4} (4 alike) : DataTypeConversion  OutDataTypeStr=double
  Discrete Derivative1 : simulink/Discrete/Discrete Derivative  gainval=1.0  ICPrevScaledInput=0.0  OutMin=[]  OutMax=[]  OutDataType=fixdt(1, 16)  OutScaling=2^-10  DoSatur=off
  Discrete-Time Integrator : DiscreteIntegrator  SampleTime=-1  LimitOutput=on  UpperSaturationLimit=1000  LowerSaturationLimit=-1000  ICPrevOutput=DiscIntNeverNeededParam  ICPrevScaledInput=DiscIntNeverNeededParam
  Product1 : Product
  Product2 : Product
  Product3 : Product
  Sum1 : Sum  Inputs=+++
  Tau : Outport
  wires:
  Product2/1 -> Discrete-Time Integrator/1
  error/1 -> Data Type Conversion1/1
  Product3/1 -> Discrete Derivative1/1
  KP/1 -> Data Type Conversion3/1
  Sum1/1 -> Tau/1
  Discrete Derivative1/1 -> Sum1/3
  Product1/1 -> Sum1/1
  Discrete-Time Integrator/1 -> Sum1/2
  KI/1 -> Data Type Conversion2/1
  KD/1 -> Data Type Conversion4/1
  Data Type Conversion3/1 -> Product1/1
  Data Type Conversion1/1 -> Product1/2, Product3/1, Product2/1
  Data Type Conversion2/1 -> Product2/2
  Data Type Conversion4/1 -> Product3/2

== system PID_SingleJoint/DynamicsController/PID_Controller/PID_Controller4 ==
  error : Inport
  KP : Inport  Port=2
  KI : Inport  Port=3
  KD : Inport  Port=4
  Data Type Conversion{1..4} (4 alike) : DataTypeConversion  OutDataTypeStr=double
  Discrete Derivative1 : simulink/Discrete/Discrete Derivative  gainval=1.0  ICPrevScaledInput=0.0  OutMin=[]  OutMax=[]  OutDataType=fixdt(1, 16)  OutScaling=2^-10  DoSatur=off
  Discrete-Time Integrator : DiscreteIntegrator  SampleTime=-1  LimitOutput=on  UpperSaturationLimit=1000  LowerSaturationLimit=-1000  ICPrevOutput=DiscIntNeverNeededParam  ICPrevScaledInput=DiscIntNeverNeededParam
  Product1 : Product
  Product2 : Product
  Product3 : Product
  Sum1 : Sum  Inputs=+++
  Tau : Outport
  wires:
  Data Type Conversion4/1 -> Product3/2
  Data Type Conversion2/1 -> Product2/2
  Data Type Conversion1/1 -> Product2/1, Product3/1, Product1/2
  Data Type Conversion3/1 -> Product1/1
  KD/1 -> Data Type Conversion4/1
  KI/1 -> Data Type Conversion2/1
  Discrete-Time Integrator/1 -> Sum1/2
  Product1/1 -> Sum1/1
  Discrete Derivative1/1 -> Sum1/3
  Sum1/1 -> Tau/1
  KP/1 -> Data Type Conversion3/1
  Product3/1 -> Discrete Derivative1/1
  error/1 -> Data Type Conversion1/1
  Product2/1 -> Discrete-Time Integrator/1

== system PID_SingleJoint/DynamicsController/PID_Controller/PID_Controller5 ==
  error : Inport
  KP : Inport  Port=2
  KI : Inport  Port=3
  KD : Inport  Port=4
  Data Type Conversion{1..4} (4 alike) : DataTypeConversion  OutDataTypeStr=double
  Discrete Derivative1 : simulink/Discrete/Discrete Derivative  gainval=1.0  ICPrevScaledInput=0.0  OutMin=[]  OutMax=[]  OutDataType=fixdt(1, 16)  OutScaling=2^-10  DoSatur=off
  Discrete-Time Integrator : DiscreteIntegrator  SampleTime=-1  LimitOutput=on  UpperSaturationLimit=1000  LowerSaturationLimit=-1000  ICPrevOutput=DiscIntNeverNeededParam  ICPrevScaledInput=DiscIntNeverNeededParam
  Product1 : Product
  Product2 : Product
  Product3 : Product
  Sum1 : Sum  Inputs=+++
  Tau : Outport
  wires:
  Data Type Conversion4/1 -> Product3/2
  Data Type Conversion2/1 -> Product2/2
  Data Type Conversion1/1 -> Product2/1, Product3/1, Product1/2
  Data Type Conversion3/1 -> Product1/1
  KD/1 -> Data Type Conversion4/1
  KI/1 -> Data Type Conversion2/1
  Discrete-Time Integrator/1 -> Sum1/2
  Product1/1 -> Sum1/1
  Discrete Derivative1/1 -> Sum1/3
  Sum1/1 -> Tau/1
  KP/1 -> Data Type Conversion3/1
  Product3/1 -> Discrete Derivative1/1
  error/1 -> Data Type Conversion1/1
  Product2/1 -> Discrete-Time Integrator/1

== system PID_SingleJoint/DynamicsController/PID_Controller/PID_Controller6 ==
  error : Inport
  KP : Inport  Port=2
  KI : Inport  Port=3
  KD : Inport  Port=4
  Data Type Conversion{1..4} (4 alike) : DataTypeConversion  OutDataTypeStr=double
  Discrete Derivative1 : simulink/Discrete/Discrete Derivative  gainval=1.0  ICPrevScaledInput=0.0  OutMin=[]  OutMax=[]  OutDataType=fixdt(1, 16)  OutScaling=2^-10  DoSatur=off
  Discrete-Time Integrator : DiscreteIntegrator  SampleTime=-1  LimitOutput=on  UpperSaturationLimit=1000  LowerSaturationLimit=-1000  ICPrevOutput=DiscIntNeverNeededParam  ICPrevScaledInput=DiscIntNeverNeededParam
  Product1 : Product
  Product2 : Product
  Product3 : Product
  Sum1 : Sum  Inputs=+++
  Tau : Outport
  wires:
  Product2/1 -> Discrete-Time Integrator/1
  error/1 -> Data Type Conversion1/1
  Product3/1 -> Discrete Derivative1/1
  KP/1 -> Data Type Conversion3/1
  Sum1/1 -> Tau/1
  Discrete Derivative1/1 -> Sum1/3
  Product1/1 -> Sum1/1
  Discrete-Time Integrator/1 -> Sum1/2
  KI/1 -> Data Type Conversion2/1
  KD/1 -> Data Type Conversion4/1
  Data Type Conversion3/1 -> Product1/1
  Data Type Conversion1/1 -> Product1/2, Product3/1, Product2/1
  Data Type Conversion2/1 -> Product2/2
  Data Type Conversion4/1 -> Product3/2

== system PID_SingleJoint/DynamicsController/关节一正弦信号发生器/Subsystem ==
  note: $e_1(t)=\theta_d(t)-\theta(t)$
  电机外转子 实际角度(rad) : Inport
  电机外转子 正弦信号的幅值 : Inport  Port=2
  Enable : EnablePort
  Product : Product
  Sum5 : Sum  Inputs=-+|
  ref_signal : dspsrcs4/Sine Wave  Amplitude=1  Frequency=Freq  Phase=0  SampleMode=Discrete  OutComplex=Real  CompMethod=Trigonometric fcn  TableSize=Speed  SampleTime=SimpleTime  SamplesPerFrame=1  ResetState=Restart at time zero  OutputFrames=on  dataType=double  wordLen=16  udDataType=sfix(16)  fracBitsMode=Best precision  numFracBits=15  OutDataTypeStr=double  LastOutDataTypeStr=double
  限幅 : Saturate  UpperLimit=pi/3  LowerLimit=0
  外转子理想 正弦信号 : Outport
  电机外转子 跟踪误差 : Outport  Port=2
  wires:
  ref_signal/1 -> Product/1
  电机外转子 正弦信号的幅值/1 -> 限幅/1
  电机外转子 实际角度(rad)/1 -> Sum5/1
  Sum5/1 -> 电机外转子 跟踪误差/1
  Product/1 -> Sum5/2, 外转子理想 正弦信号/1
  限幅/1 -> Product/2

== system PID_SingleJoint/DynamicsController/关节三正弦信号发生器/Subsystem ==
  note: $e_1(t)=\theta_d(t)-\theta(t)$
  电机外转子 实际角度(rad) : Inport
  电机外转子 正弦信号的幅值 : Inport  Port=2
  Enable : EnablePort
  Product : Product
  Sum5 : Sum  Inputs=-+|
  ref_signal : dspsrcs4/Sine Wave  Amplitude=1  Frequency=Freq  Phase=0  SampleMode=Discrete  OutComplex=Real  CompMethod=Trigonometric fcn  TableSize=Speed  SampleTime=SimpleTime  SamplesPerFrame=1  ResetState=Restart at time zero  OutputFrames=on  dataType=double  wordLen=16  udDataType=sfix(16)  fracBitsMode=Best precision  numFracBits=15  OutDataTypeStr=double  LastOutDataTypeStr=double
  限幅 : Saturate  UpperLimit=pi/3  LowerLimit=0
  外转子理想 正弦信号 : Outport
  电机外转子 跟踪误差 : Outport  Port=2
  wires:
  ref_signal/1 -> Product/1
  电机外转子 正弦信号的幅值/1 -> 限幅/1
  电机外转子 实际角度(rad)/1 -> Sum5/1
  Sum5/1 -> 电机外转子 跟踪误差/1
  Product/1 -> Sum5/2, 外转子理想 正弦信号/1
  限幅/1 -> Product/2

== system PID_SingleJoint/DynamicsController/关节二正弦信号发生器/Subsystem ==
  note: $e_1(t)=\theta_d(t)-\theta(t)$
  电机外转子 实际角度(rad) : Inport
  电机外转子 正弦信号的幅值 : Inport  Port=2
  Enable : EnablePort
  Product : Product
  Sum5 : Sum  Inputs=-+|
  ref_signal : dspsrcs4/Sine Wave  Amplitude=1  Frequency=Freq  Phase=0  SampleMode=Discrete  OutComplex=Real  CompMethod=Trigonometric fcn  TableSize=Speed  SampleTime=SimpleTime  SamplesPerFrame=1  ResetState=Restart at time zero  OutputFrames=on  dataType=double  wordLen=16  udDataType=sfix(16)  fracBitsMode=Best precision  numFracBits=15  OutDataTypeStr=double  LastOutDataTypeStr=double
  限幅 : Saturate  UpperLimit=pi/3  LowerLimit=0
  外转子理想 正弦信号 : Outport
  电机外转子 跟踪误差 : Outport  Port=2
  wires:
  限幅/1 -> Product/2
  Product/1 -> 外转子理想 正弦信号/1, Sum5/2
  Sum5/1 -> 电机外转子 跟踪误差/1
  电机外转子 实际角度(rad)/1 -> Sum5/1
  电机外转子 正弦信号的幅值/1 -> 限幅/1
  ref_signal/1 -> Product/1

== system PID_SingleJoint/DynamicsController/关节五正弦信号发生器/Subsystem ==
  note: $e_1(t)=\theta_d(t)-\theta(t)$
  电机外转子 实际角度(rad) : Inport
  电机外转子 正弦信号的幅值 : Inport  Port=2
  Enable : EnablePort
  Product : Product
  Sum5 : Sum  Inputs=-+|
  ref_signal : dspsrcs4/Sine Wave  Amplitude=1  Frequency=Freq  Phase=0  SampleMode=Discrete  OutComplex=Real  CompMethod=Trigonometric fcn  TableSize=Speed  SampleTime=SimpleTime  SamplesPerFrame=1  ResetState=Restart at time zero  OutputFrames=on  dataType=double  wordLen=16  udDataType=sfix(16)  fracBitsMode=Best precision  numFracBits=15  OutDataTypeStr=double  LastOutDataTypeStr=double
  限幅 : Saturate  UpperLimit=pi/3  LowerLimit=0
  外转子理想 正弦信号 : Outport
  电机外转子 跟踪误差 : Outport  Port=2
  wires:
  ref_signal/1 -> Product/1
  电机外转子 正弦信号的幅值/1 -> 限幅/1
  电机外转子 实际角度(rad)/1 -> Sum5/1
  Sum5/1 -> 电机外转子 跟踪误差/1
  Product/1 -> Sum5/2, 外转子理想 正弦信号/1
  限幅/1 -> Product/2

== system PID_SingleJoint/DynamicsController/关节六正弦信号发生器/Subsystem ==
  note: $e_1(t)=\theta_d(t)-\theta(t)$
  电机外转子 实际角度(rad) : Inport
  电机外转子 正弦信号的幅值 : Inport  Port=2
  Enable : EnablePort
  Product : Product
  Sum5 : Sum  Inputs=-+|
  ref_signal : dspsrcs4/Sine Wave  Amplitude=1  Frequency=Freq  Phase=0  SampleMode=Discrete  OutComplex=Real  CompMethod=Trigonometric fcn  TableSize=Speed  SampleTime=SimpleTime  SamplesPerFrame=1  ResetState=Restart at time zero  OutputFrames=on  dataType=double  wordLen=16  udDataType=sfix(16)  fracBitsMode=Best precision  numFracBits=15  OutDataTypeStr=double  LastOutDataTypeStr=double
  限幅 : Saturate  UpperLimit=pi/3  LowerLimit=0
  外转子理想 正弦信号 : Outport
  电机外转子 跟踪误差 : Outport  Port=2
  wires:
  限幅/1 -> Product/2
  Product/1 -> 外转子理想 正弦信号/1, Sum5/2
  Sum5/1 -> 电机外转子 跟踪误差/1
  电机外转子 实际角度(rad)/1 -> Sum5/1
  电机外转子 正弦信号的幅值/1 -> 限幅/1
  ref_signal/1 -> Product/1

== system PID_SingleJoint/DynamicsController/关节四正弦信号发生器/Subsystem ==
  note: $e_1(t)=\theta_d(t)-\theta(t)$
  电机外转子 实际角度(rad) : Inport
  电机外转子 正弦信号的幅值 : Inport  Port=2
  Enable : EnablePort
  Product : Product
  Sum5 : Sum  Inputs=-+|
  ref_signal : dspsrcs4/Sine Wave  Amplitude=1  Frequency=Freq  Phase=0  SampleMode=Discrete  OutComplex=Real  CompMethod=Trigonometric fcn  TableSize=Speed  SampleTime=SimpleTime  SamplesPerFrame=1  ResetState=Restart at time zero  OutputFrames=on  dataType=double  wordLen=16  udDataType=sfix(16)  fracBitsMode=Best precision  numFracBits=15  OutDataTypeStr=double  LastOutDataTypeStr=double
  限幅 : Saturate  UpperLimit=pi/3  LowerLimit=0
  外转子理想 正弦信号 : Outport
  电机外转子 跟踪误差 : Outport  Port=2
  wires:
  限幅/1 -> Product/2
  Product/1 -> 外转子理想 正弦信号/1, Sum5/2
  Sum5/1 -> 电机外转子 跟踪误差/1
  电机外转子 实际角度(rad)/1 -> Sum5/1
  电机外转子 正弦信号的幅值/1 -> 限幅/1
  ref_signal/1 -> Product/1

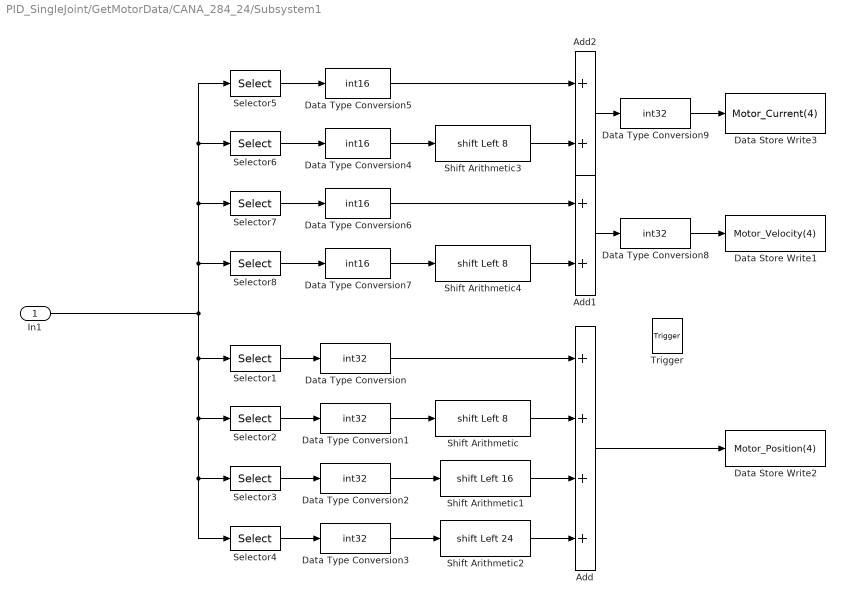
== system PID_SingleJoint/GetMotorData/CANA_284_24/Subsystem1 ==
  In1 : Inport
  Trigger : TriggerPort  TriggerType=function-call  VariantControl=Variant  PortDimensions=1
  Add : Sum  Inputs=4
  Add1 : Sum  Inputs=2
  Add2 : Sum  Inputs=2
  Data Store Write1 : DataStoreWrite  DataStoreName=Motor_Velocity  DataStoreElements=Motor_Velocity(4)
  Data Store Write2 : DataStoreWrite  DataStoreName=Motor_Position  DataStoreElements=Motor_Position(4)
  Data Store Write3 : DataStoreWrite  DataStoreName=Motor_Current  DataStoreElements=Motor_Current(4)
  Data Type Conversion{,1..3,8..9} (6 alike) : DataTypeConversion  OutDataTypeStr=int32
  Data Type Conversion{4..7} (4 alike) : DataTypeConversion  OutDataTypeStr=int16
  Selector1 : Selector  IndexMode=Zero-based  InputPortWidth=8  IndexOptions=Index vector (dialog)  Indices=4  OutputSizes=1
  Selector2 : Selector  IndexMode=Zero-based  InputPortWidth=8  IndexOptions=Index vector (dialog)  Indices=5  OutputSizes=1
  Selector3 : Selector  IndexMode=Zero-based  InputPortWidth=8  IndexOptions=Index vector (dialog)  Indices=6  OutputSizes=1
  Selector4 : Selector  IndexMode=Zero-based  InputPortWidth=8  IndexOptions=Index vector (dialog)  Indices=7  OutputSizes=1
  Selector5 : Selector  IndexMode=Zero-based  InputPortWidth=8  IndexOptions=Index vector (dialog)  Indices=0  OutputSizes=1
  Selector6 : Selector  IndexMode=Zero-based  InputPortWidth=8  IndexOptions=Index vector (dialog)  Indices=1  OutputSizes=1
  Selector7 : Selector  IndexMode=Zero-based  InputPortWidth=8  IndexOptions=Index vector (dialog)  Indices=2  OutputSizes=1
  Selector8 : Selector  IndexMode=Zero-based  InputPortWidth=8  IndexOptions=Index vector (dialog)  Indices=3  OutputSizes=1
  Shift Arithmetic : ArithShift  BitShiftNumber=8  BitShiftDirection=Left
  Shift Arithmetic1 : ArithShift  BitShiftNumber=16  BitShiftDirection=Left
  Shift Arithmetic2 : ArithShift  BitShiftNumber=24  BitShiftDirection=Left
  Shift Arithmetic3 : ArithShift  BitShiftNumber=8  BitShiftDirection=Left
  Shift Arithmetic4 : ArithShift  BitShiftNumber=8  BitShiftDirection=Left
  wires:
  Selector3/1 -> Data Type Conversion2/1
  Shift Arithmetic/1 -> Add/2
  Shift Arithmetic2/1 -> Add/4
  Data Type Conversion/1 -> Add/1
  Selector1/1 -> Data Type Conversion/1
  Selector4/1 -> Data Type Conversion3/1
  Add/1 -> Data Store Write2/1
  Shift Arithmetic1/1 -> Add/3
  Selector2/1 -> Data Type Conversion1/1
  Data Type Conversion7/1 -> Shift Arithmetic4/1
  Data Type Conversion6/1 -> Add1/1
  Selector7/1 -> Data Type Conversion6/1
  Selector8/1 -> Data Type Conversion7/1
  Selector6/1 -> Data Type Conversion4/1
  In1/1 -> Selector3/1, Selector4/1, Selector2/1, Selector1/1, Selector5/1, Selector6/1, Selector7/1, Selector8/1
  Add1/1 -> Data Type Conversion8/1
  Shift Arithmetic4/1 -> Add1/2
  Data Type Conversion1/1 -> Shift Arithmetic/1
  Data Type Conversion2/1 -> Shift Arithmetic1/1
  Data Type Conversion3/1 -> Shift Arithmetic2/1
  Selector5/1 -> Data Type Conversion5/1
  Data Type Conversion4/1 -> Shift Arithmetic3/1
  Data Type Conversion8/1 -> Data Store Write1/1
  Shift Arithmetic3/1 -> Add2/2
  Data Type Conversion5/1 -> Add2/1
  Add2/1 -> Data Type Conversion9/1
  Data Type Conversion9/1 -> Data Store Write3/1

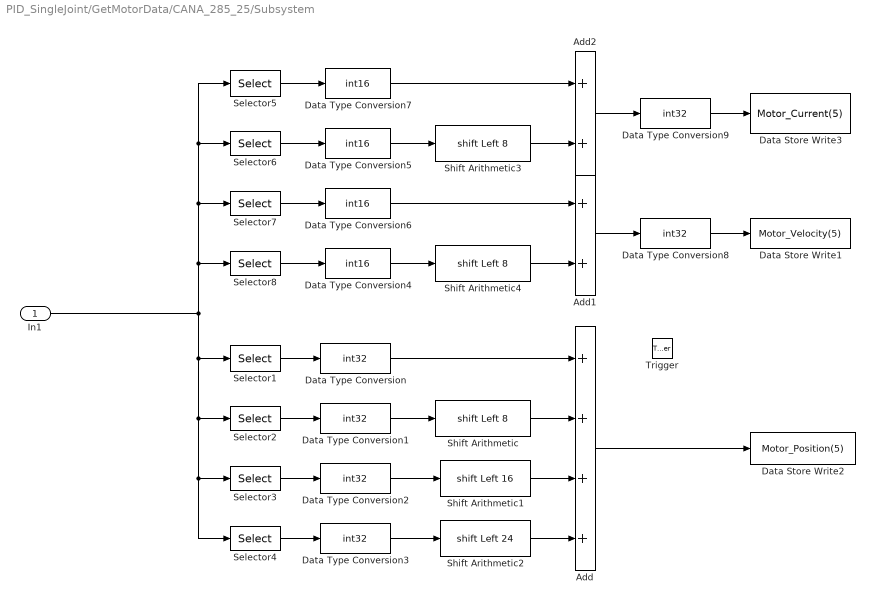
== system PID_SingleJoint/GetMotorData/CANA_285_25/Subsystem ==
  In1 : Inport
  Trigger : TriggerPort  TriggerType=function-call  VariantControl=Variant  PortDimensions=1
  Add : Sum  Inputs=4
  Add1 : Sum  Inputs=2
  Add2 : Sum  Inputs=2
  Data Store Write1 : DataStoreWrite  DataStoreName=Motor_Velocity  DataStoreElements=Motor_Velocity(5)
  Data Store Write2 : DataStoreWrite  DataStoreName=Motor_Position  DataStoreElements=Motor_Position(5)
  Data Store Write3 : DataStoreWrite  DataStoreName=Motor_Current  DataStoreElements=Motor_Current(5)
  Data Type Conversion{,1..3,8..9} (6 alike) : DataTypeConversion  OutDataTypeStr=int32
  Data Type Conversion{4..7} (4 alike) : DataTypeConversion  OutDataTypeStr=int16
  Selector1 : Selector  IndexMode=Zero-based  InputPortWidth=8  IndexOptions=Index vector (dialog)  Indices=4  OutputSizes=1
  Selector2 : Selector  IndexMode=Zero-based  InputPortWidth=8  IndexOptions=Index vector (dialog)  Indices=5  OutputSizes=1
  Selector3 : Selector  IndexMode=Zero-based  InputPortWidth=8  IndexOptions=Index vector (dialog)  Indices=6  OutputSizes=1
  Selector4 : Selector  IndexMode=Zero-based  InputPortWidth=8  IndexOptions=Index vector (dialog)  Indices=7  OutputSizes=1
  Selector5 : Selector  IndexMode=Zero-based  InputPortWidth=8  IndexOptions=Index vector (dialog)  Indices=0  OutputSizes=1
  Selector6 : Selector  IndexMode=Zero-based  InputPortWidth=8  IndexOptions=Index vector (dialog)  Indices=1  OutputSizes=1
  Selector7 : Selector  IndexMode=Zero-based  InputPortWidth=8  IndexOptions=Index vector (dialog)  Indices=2  OutputSizes=1
  Selector8 : Selector  IndexMode=Zero-based  InputPortWidth=8  IndexOptions=Index vector (dialog)  Indices=3  OutputSizes=1
  Shift Arithmetic : ArithShift  BitShiftNumber=8  BitShiftDirection=Left
  Shift Arithmetic1 : ArithShift  BitShiftNumber=16  BitShiftDirection=Left
  Shift Arithmetic2 : ArithShift  BitShiftNumber=24  BitShiftDirection=Left
  Shift Arithmetic3 : ArithShift  BitShiftNumber=8  BitShiftDirection=Left
  Shift Arithmetic4 : ArithShift  BitShiftNumber=8  BitShiftDirection=Left
  wires:
  Selector3/1 -> Data Type Conversion2/1
  Shift Arithmetic/1 -> Add/2
  Shift Arithmetic2/1 -> Add/4
  Data Type Conversion/1 -> Add/1
  Selector1/1 -> Data Type Conversion/1
  Selector4/1 -> Data Type Conversion3/1
  Add/1 -> Data Store Write2/1
  Shift Arithmetic1/1 -> Add/3
  Selector2/1 -> Data Type Conversion1/1
  Selector5/1 -> Data Type Conversion7/1
  Selector8/1 -> Data Type Conversion4/1
  Data Type Conversion4/1 -> Shift Arithmetic4/1
  Data Type Conversion6/1 -> Add1/1
  Selector7/1 -> Data Type Conversion6/1
  Selector6/1 -> Data Type Conversion5/1
  In1/1 -> Selector3/1, Selector4/1, Selector2/1, Selector1/1, Selector5/1, Selector6/1, Selector7/1, Selector8/1
  Add1/1 -> Data Type Conversion8/1
  Data Type Conversion1/1 -> Shift Arithmetic/1
  Data Type Conversion2/1 -> Shift Arithmetic1/1
  Data Type Conversion3/1 -> Shift Arithmetic2/1
  Data Type Conversion5/1 -> Shift Arithmetic3/1
  Shift Arithmetic4/1 -> Add1/2
  Shift Arithmetic3/1 -> Add2/2
  Data Type Conversion7/1 -> Add2/1
  Add2/1 -> Data Type Conversion9/1
  Data Type Conversion8/1 -> Data Store Write1/1
  Data Type Conversion9/1 -> Data Store Write3/1
